simulink model "Circuit2_v5_2018b"  (R2018b)
settings: Solver=ode4  StartTime=0.0  StopTime=5  FixedStep=1e-4  RelTol=1e-3
values from neighbouring files (symbols this model uses):
  Be = 1300e6    (= 1300000000)    [Circuit1_load.m]    (also in Circuit2_values.m)
  BeA = 1200e6    (= 1200000000)    [Circuit2_values.m]    (also in Circut3_values.m = 1300000000)
  BeB = 1500e6    (= 1500000000)    [Circuit2_values.m]    (also in Circut3_values.m = 1300000000)
  Cd = 0.7    [Circuit1_load.m]    (also in Circuit2_values.m)
  Dorifice = 2e-2    (= 0.02)    [Circuit1_load.m]    (also in Circuit2_values.m = 0.004)
  Dspool = 1e-2    (= 0.01)    [Circuit2_values.m]
  Kp = (1.e-3)/(10e5)    (= 1e-09)    [Circuit1_load.m]    (also in Circuit2_values.m; Circut3_values.m)
  pA0 = 1e5    (= 100000)    [Circuit2_values.m]    (also in Circut3_values.m = 7300000)
  pB0 = 1e5    (= 100000)    [Circuit2_values.m]    (also in Circut3_values.m = 700000)
  pp0 = 180e5    (= 18000000)    [Circuit2_values.m]
  pref = 180e5    (= 18000000)    [Circuit1_load.m]    (also in Circuit2_values.m; Circut3_values.m = 17000000)
  rho = 860    [Circuit1_load.m]    (also in Circuit2_values.m; Circut3_values.m)
  tau = 60e-3    (= 0.06)    [Circuit1_load.m]    (also in Circuit2_values.m = 0.03)
  V = 3e-3    (= 0.003)    [Circuit1_load.m]    (also in Circuit2_values.m)
  VA = 5e-4    (= 0.0005)    [Circuit2_values.m]    (also in Circut3_values.m = 0.0015)
  VB = 5e-4    (= 0.0005)    [Circuit2_values.m]    (also in Circut3_values.m = 0.003)
undefined symbols (not defined in the file or in its folder): sgn
settings Model: Creator=Janne  LastModifiedBy=Alex

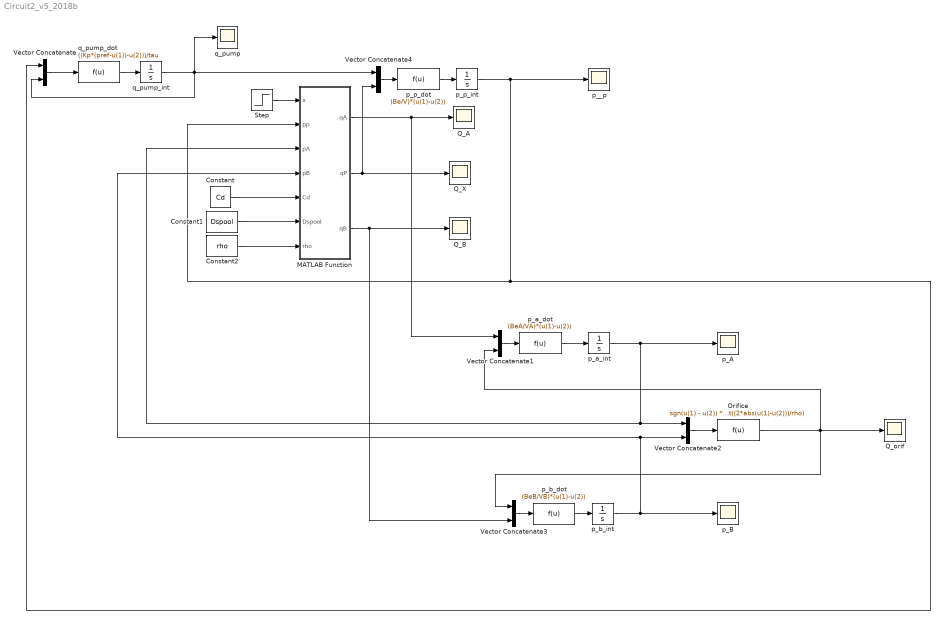
== system Circuit2_v5_2018b ==
  Constant : Constant  Value=Cd
  Constant1 : Constant  Value=Dspool
  Constant2 : Constant  Value=rho
  MATLAB Function : MATLAB Function  TreatAsAtomicUnit=on
  Orifice : Fcn  Expr=sgn(u(1) - u(2)) *Cd*(1/4 * pi * Dorifice^2)*sqrt((2*abs(u(1)-u(2)))/rho)
  Q_A : Scope
  Q_B : Scope
  Q_X : Scope
  Q_orif : Scope
  Step : Step  Time=2  Before=-0.0004  After=0.0004  SampleTime=0
  Vector Concatenate{,1..4} (5 alike) : Concatenate
  p_A : Scope
  p_B : Scope
  p__p : Scope
  p_a_dot : Fcn  Expr=(BeA/VA)*(u(1)-u(2))
  p_a_int : Integrator  InitialCondition=pA0  LimitOutput=on  UpperSaturationLimit=1000e5  LowerSaturationLimit=0
  p_b_dot : Fcn  Expr=(BeB/VB)*(u(1)-u(2))
  p_b_int : Integrator  InitialCondition=pB0  LimitOutput=on  UpperSaturationLimit=1000e5  LowerSaturationLimit=0
  p_p_dot : Fcn  Expr=(Be/V)*(u(1)-u(2))
  p_p_int : Integrator  InitialCondition=pp0  LimitOutput=on  UpperSaturationLimit=1000e5  LowerSaturationLimit=0
  q_pump : Scope
  q_pump_dot : Fcn  Expr=((Kp*(pref-u(1))-u(2)))/tau
  q_pump_int : Integrator  LimitOutput=on  UpperSaturationLimit=1000e5  LowerSaturationLimit=0
  wires:
  q_pump_dot/1 -> q_pump_int/1
  Vector Concatenate/1 -> q_pump_dot/1
  q_pump_int/1 -> q_pump/1, Vector Concatenate/2, Vector Concatenate4/1
  Vector Concatenate4/1 -> p_p_dot/1
  p_p_dot/1 -> p_p_int/1
  Step/1 -> MATLAB Function/1(x)
  p_p_int/1 -> Vector Concatenate/1, MATLAB Function/2(pp), p__p/1
  Constant/1 -> MATLAB Function/5(Cd)
  Constant1/1 -> MATLAB Function/6(Dspool)
  Constant2/1 -> MATLAB Function/7(rho)
  p_a_dot/1 -> p_a_int/1
  p_b_dot/1 -> p_b_int/1
  Vector Concatenate1/1 -> p_a_dot/1
  Vector Concatenate3/1 -> p_b_dot/1
  p_a_int/1 -> p_A/1, MATLAB Function/3(pA), Vector Concatenate2/1
  MATLAB Function/1(qA) -> Vector Concatenate1/1, Q_A/1
  Vector Concatenate2/1 -> Orifice/1
  p_b_int/1 -> MATLAB Function/4(pB), Vector Concatenate2/2, p_B/1
  MATLAB Function/2(qP) -> Q_X/1, Vector Concatenate4/2
  MATLAB Function/3(qB) -> Vector Concatenate3/2, Q_B/1
  Orifice/1 -> Vector Concatenate3/1, Q_orif/1, Vector Concatenate1/2

== matlab function Circuit2_v5_2018b/MATLAB Function ==
  data: x input; pp input; pA input; pB input; qA output; Cd input; Dspool input; rho input; qP output; qB output
function [qA,qP,qB] = fcn(x, pp, pA, pB, Cd, Dspool, rho)
 
 qA = 0;

 qB = 0;

 qP = 0;
 
 if x >= 0
     qA = Cd*pi*Dspool*x*sqrt(2*abs(pp-pA)/rho)*sign(pp-pA);

     qB = Cd*pi*Dspool*x*sqrt(2*pB/rho);

     qP = qA;
 else
    qB = Cd*pi*Dspool*x*sqrt(2*abs(pp-pB)/rho)*sign(pp-pB);

    qA = Cd*pi*Dspool*x*sqrt(2*pA/rho);
    
    qP = -qB;
 end
